simulink model "ex2"  (R2022a)
settings: Solver=VariableStepAuto  StartTime=1  StopTime=10.0  RelTol=1e-3
settings Model: Creator=loryb  LastModifiedBy=loryb
settings DataIOCC: LimitDataPoints=on  SaveFinalState=on  SaveOperatingPoint=on

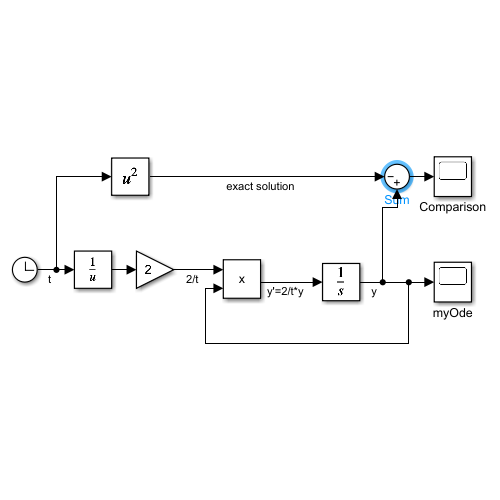
[thumbnail: Simulink's stored preview of the top-level diagram]
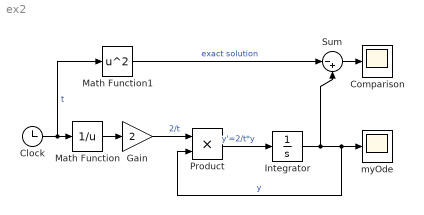
== system ex2 ==
  Clock : Clock
  Comparison : Scope
  Gain : Gain  Gain=2
  Integrator : Integrator  InitialCondition=1
  Math Function : Math  Operator=reciprocal
  Math Function1 : Math  Operator=square
  Product : Product
  Sum : Sum  Inputs=|-+
  myOde : Scope
  wires:
  Clock/1 -> Math Function1/1, Math Function/1  "t"
  Math Function/1 -> Gain/1
  Gain/1 -> Product/1  "2/t"
  Product/1 -> Integrator/1  "y'=2/t*y"
  Integrator/1 -> Product/2, myOde/1, Sum/2  "y"
  Math Function1/1 -> Sum/1  "exact solution"
  Sum/1 -> Comparison/1
